simulink model "game_example"  (R2020b)
settings: Solver=ode4  StartTime=0.0  StopTime=tstop  FixedStep=0.01  RelTol=1e-3
values from neighbouring files (symbols this model uses):
  c = 0.25    [main.m]
  K = [1;0.5]    [main.m]
  N = 4    [main.m]
  ubar = [-4,-12,1,16 ... (first row only)    [main.m]
  umax = [10;6]    [main.m]
  umin = [-5;-6]    [main.m]
  x0 = zeros(nx,N)    [main.m]    (also in simulation_test.m = [0.1;0.1;pi/2])
settings Model: Creator=dliaomcp  LastModifiedBy=dliaomcp
settings DebuggingCC: UnderSpecifiedDimensionMsg=warning

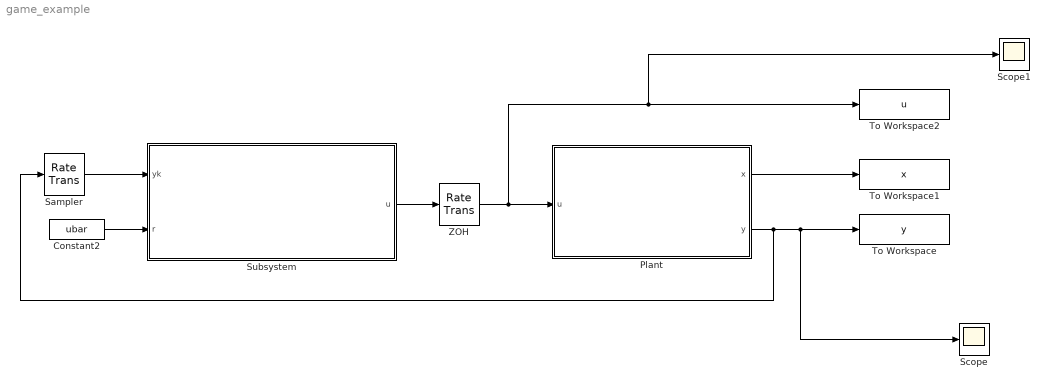
== system game_example ==
  Constant2 : Constant  Value=ubar
  Plant : Subsystem
  Sampler : RateTransition  OutPortSampleTime=ts
  Scope : Scope
  Scope1 : Scope
  Subsystem : Subsystem
  To Workspace : ToWorkspace  VariableName=y  SaveFormat=Timeseries  SampleTime=-1
  To Workspace1 : ToWorkspace  VariableName=x  SaveFormat=Timeseries  SampleTime=-1
  To Workspace2 : ToWorkspace  VariableName=u  SaveFormat=Timeseries  SampleTime=-1
  ZOH : RateTransition  InitialCondition=zeros(2,N)  OutPortSampleTimeOpt=Inherit
  wires:
  Sampler/1 -> Subsystem/1(yk)
  Subsystem/1(u) -> ZOH/1
  ZOH/1 -> Scope1/1, To Workspace2/1, Plant/1(u)
  Constant2/1 -> Subsystem/2(r)
  Plant/2(y) -> Sampler/1, Scope/1, To Workspace/1
  Plant/1(x) -> To Workspace1/1

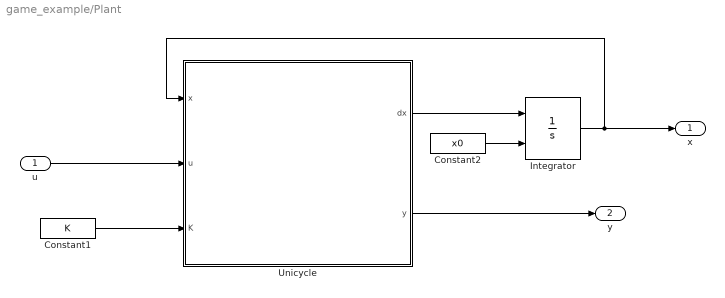
== system game_example/Plant ==
  u : Inport
  Constant1 : Constant  Value=K
  Constant2 : Constant  Value=x0
  Integrator : Integrator  InitialConditionSource=external
  Unicycle : MATLAB Function  TreatAsAtomicUnit=on
  x : Outport
  y : Outport  Port=2
  wires:
  Unicycle/2(y) -> y/1
  Unicycle/1(dx) -> Integrator/1
  Constant1/1 -> Unicycle/3(K)
  u/1 -> Unicycle/2(u)
  Constant2/1 -> Integrator/2
  Integrator/1 -> x/1, Unicycle/1(x)

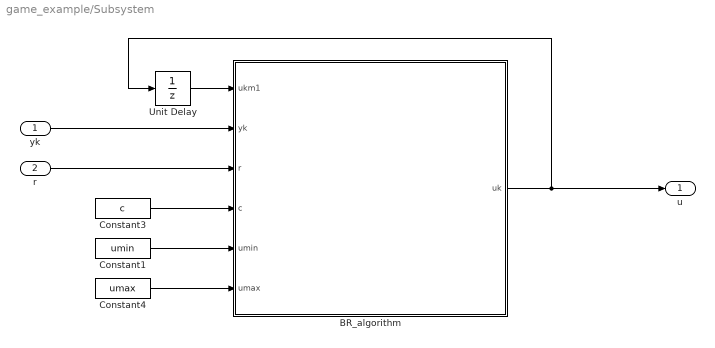
== system game_example/Subsystem ==
  yk : Inport
  r : Inport  Port=2
  BR_algorithm : MATLAB Function  TreatAsAtomicUnit=on
  Constant1 : Constant  Value=umin
  Constant3 : Constant  Value=c
  Constant4 : Constant  Value=umax
  Unit Delay : UnitDelay  InitialCondition=zeros(2,N)  SampleTime=-1  HasFrameUpgradeWarning=on
  u : Outport
  wires:
  Constant1/1 -> BR_algorithm/5(umin)
  BR_algorithm/1(uk) -> u/1, Unit Delay/1
  yk/1 -> BR_algorithm/2(yk)
  Constant4/1 -> BR_algorithm/6(umax)
  Unit Delay/1 -> BR_algorithm/1(ukm1)
  Constant3/1 -> BR_algorithm/4(c)
  r/1 -> BR_algorithm/3(r)

== matlab function game_example/Subsystem/BR_algorithm ==
  data: ukm1 input; uk output; yk input; r input; c input; umin input; umax input; N parameter
function uk = feedback_best_response(ukm1,yk,r,c,umin,umax,N)


uk = zeros(2,N);

coder.extrinsic('best_response');
for j = 1:N
    uk(:,j) = best_response(r(:,j),yk,j,c,umax,umin);
end

end

== matlab function game_example/Plant/Unicycle ==
  data: x input; dx output; u input; y output; K input; N parameter
function [dx,y] = plant(x,u,K,N)
    dx = zeros(3,N);
    y = zeros(2,N);
    for j = 1:N
        [dx(:,j),y(:,j)] = agent_dynamics(x(:,j),u(:,j),K);
    end
end
